simulink model "Navneet_1458_Day_4"  (R2025b)
settings: Solver=VariableStepAuto  StartTime=0.0  StopTime=10.0  RelTol=1e-3
settings Model: Creator=AUTBLT509  LastModifiedBy=AUTBLT509

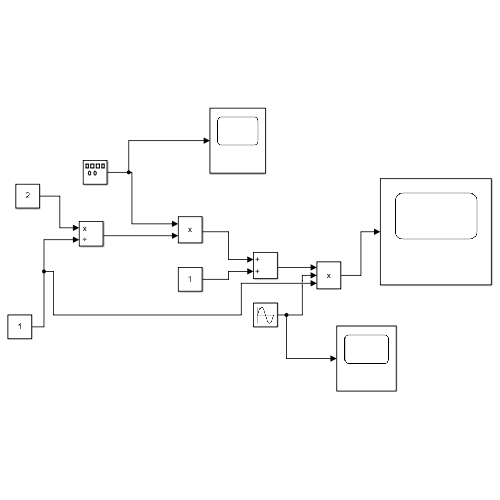
[thumbnail: Simulink's stored preview of the top-level diagram]
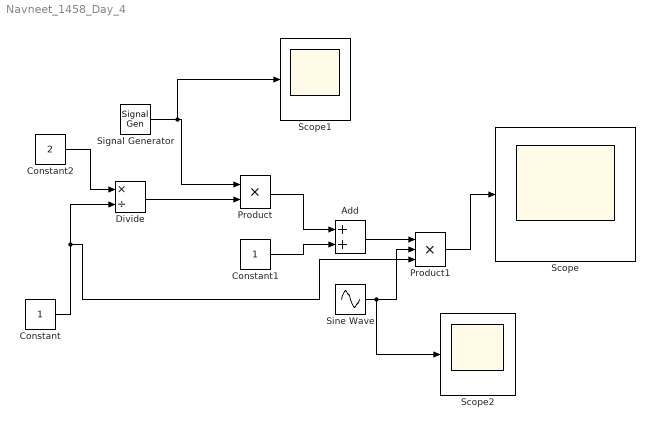
== system Navneet_1458_Day_4 ==
  Add : Sum
  Constant : Constant
  Constant1 : Constant
  Constant2 : Constant  Value=2
  Divide : Product  Inputs=*/
  Product : Product
  Product1 : Product  Inputs=3
  Scope : Scope
      settings: ActiveDisplayYMinimum=-8.09748310323405  ActiveDisplayYMaximum=8.584060125713135
  Scope1 : Scope
      settings: ActiveDisplayYMinimum=-2.6946389256547181  ActiveDisplayYMaximum=6.15193961036842
  Scope2 : Scope
      settings: ActiveDisplayYMinimum=-5.4977020771779834  ActiveDisplayYMaximum=2.1443050806003425  DataLoggingVariableName=ScopeData2
  Signal Generator : SignalGenerator  WaveForm=square  Frequency=10  Units=rad/sec
  Sine Wave : Sin  Frequency=100  SampleTime=0
  wires:
  Constant/1 -> Divide/2, Product1/3
  Constant2/1 -> Divide/1
  Divide/1 -> Product/2
  Constant1/1 -> Add/2
  Product/1 -> Add/1
  Add/1 -> Product1/1
  Sine Wave/1 -> Product1/2, Scope2/1
  Product1/1 -> Scope/1
  Signal Generator/1 -> Scope1/1, Product/1
